simulink model "TST_FlWtDet_DD"  (R2016b)
settings: Solver=FixedStepDiscrete  StartTime=0.0  StopTime=simTime  FixedStep=sampleTime  RelTol=1e-3
values from neighbouring files (symbols this model uses):
  testCase = 1    [initTST_FlWtDet_DD_001.m]    (also in initTST_FlWtDet_DD_002.m = 2)
libraries: simulink x5, UnitTest_Lib x2
settings Model: Creator=zhengjinyan  LastModifiedBy=zhengjinyan
settings DebuggingCC: SignalRangeChecking=error

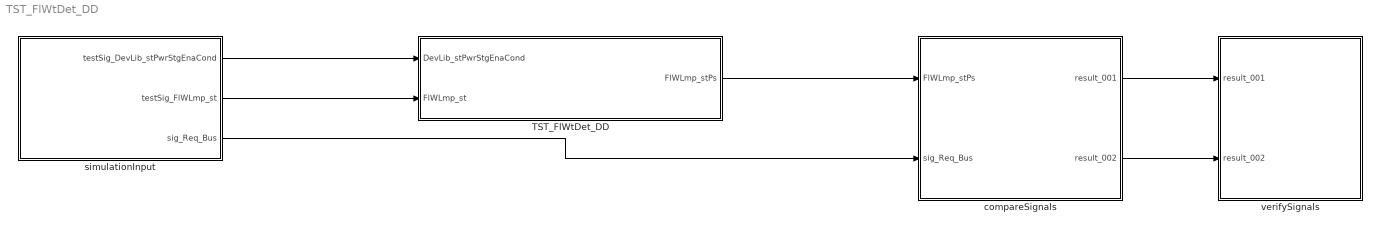
== system TST_FlWtDet_DD ==
  TST_FlWtDet_DD : Subsystem
  compareSignals : Subsystem
  simulationInput : Subsystem
  verifySignals : Subsystem
  wires:
  simulationInput/1(testSig_DevLib_stPwrStgEnaCond) -> TST_FlWtDet_DD/1(DevLib_stPwrStgEnaCond)
  simulationInput/2(testSig_FlWLmp_st) -> TST_FlWtDet_DD/2(FlWLmp_st)
  TST_FlWtDet_DD/1(FlWLmp_stPs) -> compareSignals/1(FlWLmp_stPs)
  simulationInput/3(sig_Req_Bus) -> compareSignals/2(sig_Req_Bus)
  compareSignals/1(result_001) -> verifySignals/1(result_001)
  compareSignals/2(result_002) -> verifySignals/2(result_002)

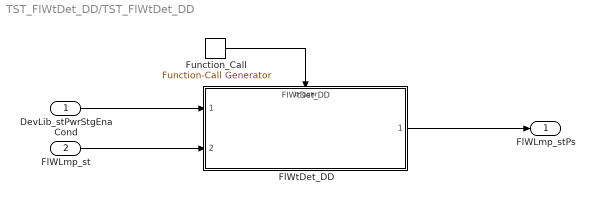
== system TST_FlWtDet_DD/TST_FlWtDet_DD ==
  DevLib_stPwrStgEnaCond : Inport
  FlWLmp_st : Inport  Port=2
  FlWtDet_DD : ModelReference  ModelNameDialog=FlWtDet_DD  SimulationMode=Normal  ModelReferenceVersion=1.8  TriggerPortName=function  TriggerPortTriggerType=function-call  TriggerPortStatesWhenEnabling=held
  Function_Call : simulink/Ports & Subsystems/Function-Call Generator  sample_time=sampleTime  numberOfIterations=1
  FlWLmp_stPs : Outport
  wires:
  Function_Call/1 -> FlWtDet_DD/Trigger
  DevLib_stPwrStgEnaCond/1 -> FlWtDet_DD/1
  FlWLmp_st/1 -> FlWtDet_DD/2
  FlWtDet_DD/1 -> FlWLmp_stPs/1

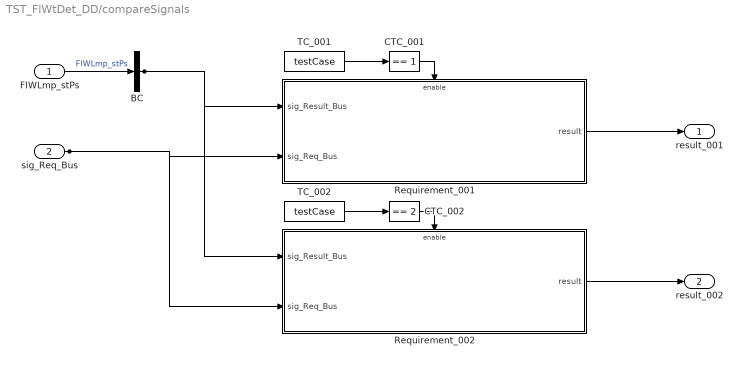
== system TST_FlWtDet_DD/compareSignals ==
  FlWLmp_stPs : Inport
  sig_Req_Bus : Inport  Port=2
  BC : BusCreator  Inputs=1
  CTC_001 : simulink/Logic and Bit Operations/Compare To Constant  relop===  const=1  OutDataTypeStr=boolean
  CTC_002 : simulink/Logic and Bit Operations/Compare To Constant  relop===  const=2  OutDataTypeStr=boolean
  Requirement_001 : Subsystem
  Requirement_002 : Subsystem
  TC_001 : Constant  Value=testCase
  TC_002 : Constant  Value=testCase
  result_001 : Outport
  result_002 : Outport  Port=2
  wires:
  FlWLmp_stPs/1 -> BC/1  "FlWLmp_stPs"
  TC_001/1 -> CTC_001/1
  CTC_001/1 -> Requirement_001/Enable
  sig_Req_Bus/1 -> Requirement_001/2(sig_Req_Bus), Requirement_002/2(sig_Req_Bus)
  BC/1 -> Requirement_001/1(sig_Result_Bus), Requirement_002/1(sig_Result_Bus)
  Requirement_001/1(result) -> result_001/1
  TC_002/1 -> CTC_002/1
  CTC_002/1 -> Requirement_002/Enable
  Requirement_002/1(result) -> result_002/1

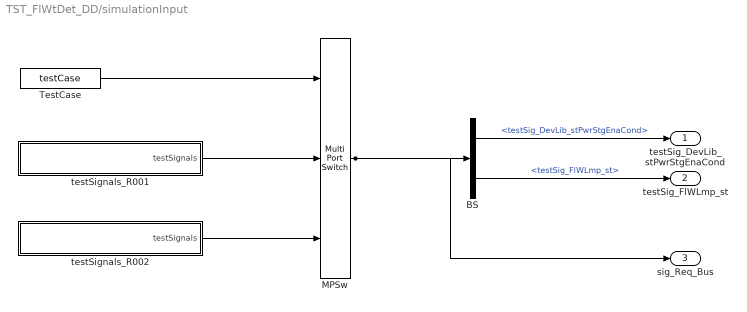
== system TST_FlWtDet_DD/simulationInput ==
  BS : BusSelector  OutputSignals=testSig_DevLib_stPwrStgEnaCond,testSig_FlWLmp_st
  MPSw : MultiPortSwitch  Inputs=2  SaturateOnIntegerOverflow=on  InputSameDT=on
  TestCase : Constant  Value=testCase
  testSignals_R001 : Subsystem
  testSignals_R002 : Subsystem
  testSig_DevLib_stPwrStgEnaCond : Outport
  testSig_FlWLmp_st : Outport  Port=2
  sig_Req_Bus : Outport  Port=3
  wires:
  BS/1 -> testSig_DevLib_stPwrStgEnaCond/1  "<testSig_DevLib_stPwrStgEnaCond>"
  BS/2 -> testSig_FlWLmp_st/1  "<testSig_FlWLmp_st>"
  MPSw/1 -> BS/1, sig_Req_Bus/1
  TestCase/1 -> MPSw/1
  testSignals_R001/1(testSignals) -> MPSw/2
  testSignals_R002/1(testSignals) -> MPSw/3

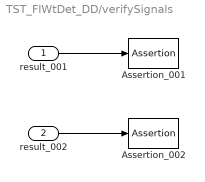
== system TST_FlWtDet_DD/verifySignals ==
  result_001 : Inport
  result_002 : Inport  Port=2
  Assertion_001 : Assertion  Enabled=off
  Assertion_002 : Assertion  Enabled=off
  wires:
  result_001/1 -> Assertion_001/1
  result_002/1 -> Assertion_002/1

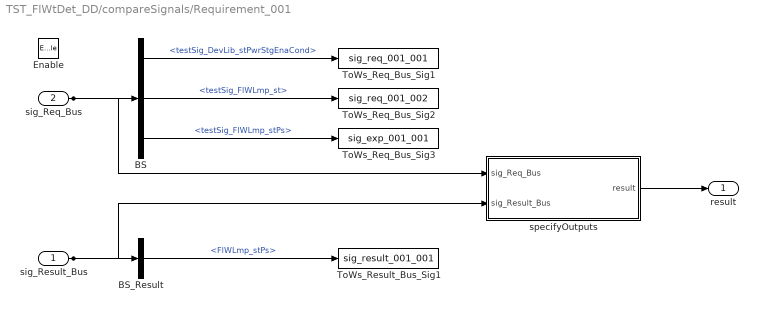
== system TST_FlWtDet_DD/compareSignals/Requirement_001 ==
  sig_Result_Bus : Inport
  sig_Req_Bus : Inport  Port=2
  Enable : EnablePort
  BS : BusSelector  OutputSignals=testSig_DevLib_stPwrStgEnaCond,testSig_FlWLmp_st,testSig_FlWLmp_stPs
  BS_Result : BusSelector  OutputSignals=FlWLmp_stPs
  ToWs_Req_Bus_Sig1 : ToWorkspace  VariableName=sig_req_001_001  SaveFormat=Structure With Time
  ToWs_Req_Bus_Sig2 : ToWorkspace  VariableName=sig_req_001_002  SaveFormat=Structure With Time
  ToWs_Req_Bus_Sig3 : ToWorkspace  VariableName=sig_exp_001_001  SaveFormat=Structure With Time
  ToWs_Result_Bus_Sig1 : ToWorkspace  VariableName=sig_result_001_001  SaveFormat=Structure With Time
  specifyOutputs : Subsystem
  result : Outport
  wires:
  sig_Req_Bus/1 -> BS/1, specifyOutputs/1(sig_Req_Bus)
  BS/1 -> ToWs_Req_Bus_Sig1/1  "<testSig_DevLib_stPwrStgEnaCond>"
  BS/2 -> ToWs_Req_Bus_Sig2/1  "<testSig_FlWLmp_st>"
  BS/3 -> ToWs_Req_Bus_Sig3/1  "<testSig_FlWLmp_stPs>"
  sig_Result_Bus/1 -> BS_Result/1, specifyOutputs/2(sig_Result_Bus)
  BS_Result/1 -> ToWs_Result_Bus_Sig1/1  "<FlWLmp_stPs>"
  specifyOutputs/1(result) -> result/1

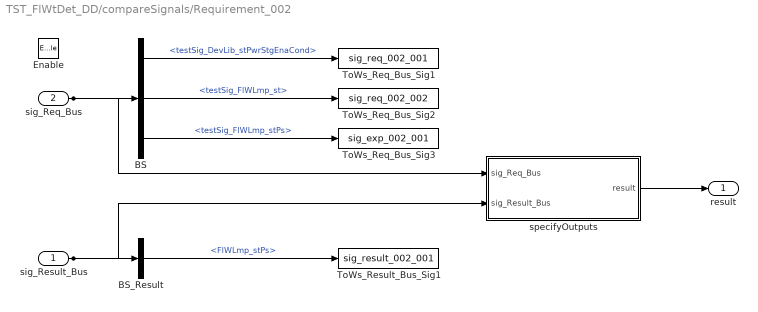
== system TST_FlWtDet_DD/compareSignals/Requirement_002 ==
  sig_Result_Bus : Inport
  sig_Req_Bus : Inport  Port=2
  Enable : EnablePort
  BS : BusSelector  OutputSignals=testSig_DevLib_stPwrStgEnaCond,testSig_FlWLmp_st,testSig_FlWLmp_stPs
  BS_Result : BusSelector  OutputSignals=FlWLmp_stPs
  ToWs_Req_Bus_Sig1 : ToWorkspace  VariableName=sig_req_002_001  SaveFormat=Structure With Time
  ToWs_Req_Bus_Sig2 : ToWorkspace  VariableName=sig_req_002_002  SaveFormat=Structure With Time
  ToWs_Req_Bus_Sig3 : ToWorkspace  VariableName=sig_exp_002_001  SaveFormat=Structure With Time
  ToWs_Result_Bus_Sig1 : ToWorkspace  VariableName=sig_result_002_001  SaveFormat=Structure With Time
  specifyOutputs : Subsystem
  result : Outport
  wires:
  sig_Req_Bus/1 -> BS/1, specifyOutputs/1(sig_Req_Bus)
  BS/1 -> ToWs_Req_Bus_Sig1/1  "<testSig_DevLib_stPwrStgEnaCond>"
  BS/2 -> ToWs_Req_Bus_Sig2/1  "<testSig_FlWLmp_st>"
  BS/3 -> ToWs_Req_Bus_Sig3/1  "<testSig_FlWLmp_stPs>"
  sig_Result_Bus/1 -> BS_Result/1, specifyOutputs/2(sig_Result_Bus)
  BS_Result/1 -> ToWs_Result_Bus_Sig1/1  "<FlWLmp_stPs>"
  specifyOutputs/1(result) -> result/1

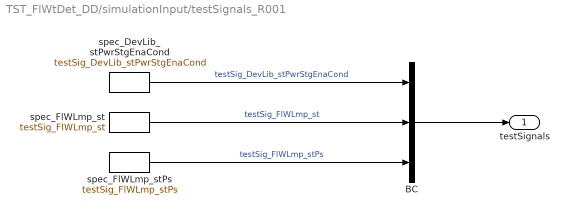
== system TST_FlWtDet_DD/simulationInput/testSignals_R001 ==
  BC : BusCreator  Inputs=3
  spec_DevLib_stPwrStgEnaCond : FromWorkspace  VariableName=testSig_DevLib_stPwrStgEnaCond  Interpolate=off  OutputAfterFinalValue=Holding final value
  spec_FlWLmp_st : FromWorkspace  VariableName=testSig_FlWLmp_st  Interpolate=off  OutputAfterFinalValue=Holding final value
  spec_FlWLmp_stPs : FromWorkspace  VariableName=testSig_FlWLmp_stPs  Interpolate=off  OutputAfterFinalValue=Holding final value
  testSignals : Outport
  wires:
  BC/1 -> testSignals/1
  spec_DevLib_stPwrStgEnaCond/1 -> BC/1  "testSig_DevLib_stPwrStgEnaCond"
  spec_FlWLmp_st/1 -> BC/2  "testSig_FlWLmp_st"
  spec_FlWLmp_stPs/1 -> BC/3  "testSig_FlWLmp_stPs"

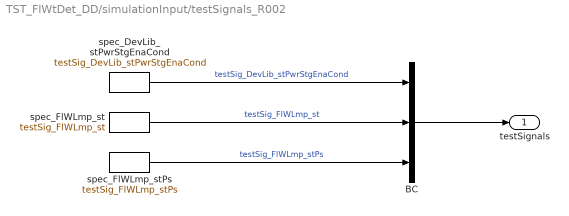
== system TST_FlWtDet_DD/simulationInput/testSignals_R002 ==
  BC : BusCreator  Inputs=3
  spec_DevLib_stPwrStgEnaCond : FromWorkspace  VariableName=testSig_DevLib_stPwrStgEnaCond  Interpolate=off  OutputAfterFinalValue=Holding final value
  spec_FlWLmp_st : FromWorkspace  VariableName=testSig_FlWLmp_st  Interpolate=off  OutputAfterFinalValue=Holding final value
  spec_FlWLmp_stPs : FromWorkspace  VariableName=testSig_FlWLmp_stPs  Interpolate=off  OutputAfterFinalValue=Holding final value
  testSignals : Outport
  wires:
  BC/1 -> testSignals/1
  spec_DevLib_stPwrStgEnaCond/1 -> BC/1  "testSig_DevLib_stPwrStgEnaCond"
  spec_FlWLmp_st/1 -> BC/2  "testSig_FlWLmp_st"
  spec_FlWLmp_stPs/1 -> BC/3  "testSig_FlWLmp_stPs"

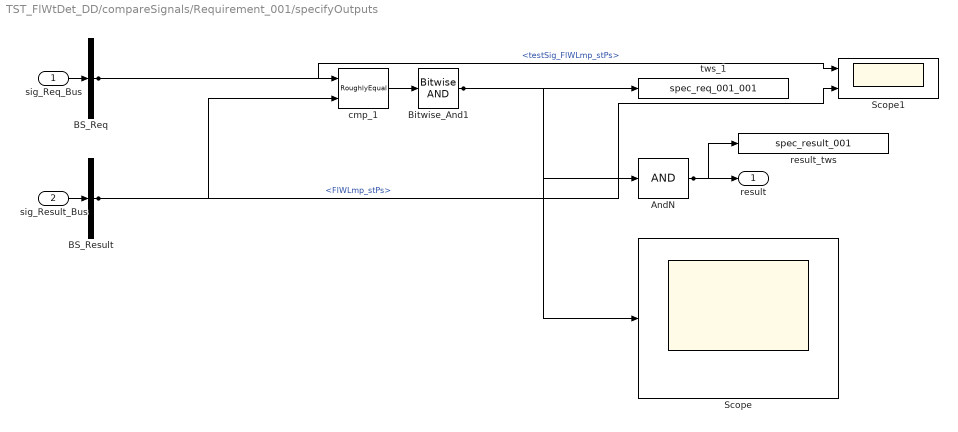
== system TST_FlWtDet_DD/compareSignals/Requirement_001/specifyOutputs ==
  sig_Req_Bus : Inport
  sig_Result_Bus : Inport  Port=2
  AndN : Logic  Inputs=1
  BS_Req : BusSelector  OutputSignals=testSig_FlWLmp_stPs
  BS_Result : BusSelector  OutputSignals=FlWLmp_stPs
  Bitwise_And1 : simulink/Logic and Bit Operations/Bitwise Operator  logicop=AND  UseBitMask=off  BitMask=bin2dec('11011001')  BitMaskRealWorld=Stored Integer
  Scope : Scope
  Scope1 : Scope  NumInputPorts=2
  cmp_1 : UnitTest_Lib/RoughlyEqual  slope=0.1
  result_tws : ToWorkspace  VariableName=spec_result_001
  tws_1 : ToWorkspace  VariableName=spec_req_001_001
  result : Outport
  wires:
  sig_Req_Bus/1 -> BS_Req/1
  sig_Result_Bus/1 -> BS_Result/1
  AndN/1 -> result/1, result_tws/1
  BS_Req/1 -> cmp_1/1, Scope1/1  "<testSig_FlWLmp_stPs>"
  BS_Result/1 -> cmp_1/2, Scope1/2  "<FlWLmp_stPs>"
  cmp_1/1 -> Bitwise_And1/1
  Bitwise_And1/1 -> tws_1/1, AndN/1, Scope/1

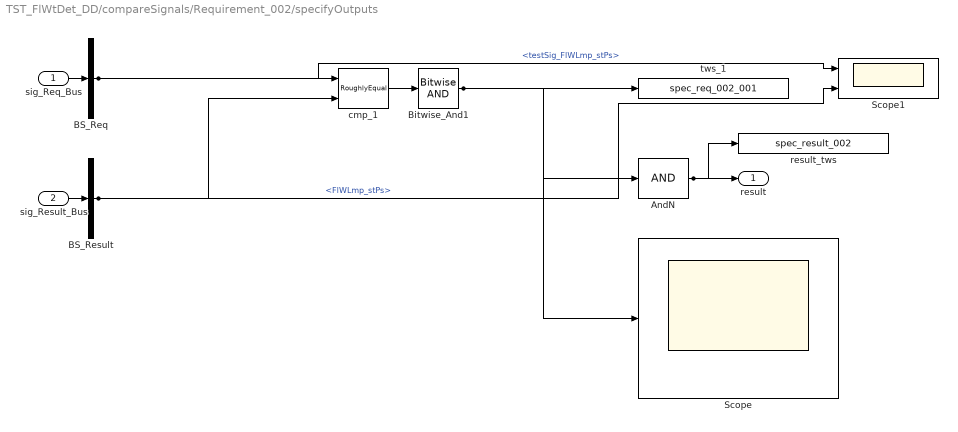
== system TST_FlWtDet_DD/compareSignals/Requirement_002/specifyOutputs ==
  sig_Req_Bus : Inport
  sig_Result_Bus : Inport  Port=2
  AndN : Logic  Inputs=1
  BS_Req : BusSelector  OutputSignals=testSig_FlWLmp_stPs
  BS_Result : BusSelector  OutputSignals=FlWLmp_stPs
  Bitwise_And1 : simulink/Logic and Bit Operations/Bitwise Operator  logicop=AND  UseBitMask=off  BitMask=bin2dec('11011001')  BitMaskRealWorld=Stored Integer
  Scope : Scope
  Scope1 : Scope  NumInputPorts=2
  cmp_1 : UnitTest_Lib/RoughlyEqual  slope=0.1
  result_tws : ToWorkspace  VariableName=spec_result_002
  tws_1 : ToWorkspace  VariableName=spec_req_002_001
  result : Outport
  wires:
  sig_Req_Bus/1 -> BS_Req/1
  sig_Result_Bus/1 -> BS_Result/1
  AndN/1 -> result/1, result_tws/1
  BS_Req/1 -> cmp_1/1, Scope1/1  "<testSig_FlWLmp_stPs>"
  BS_Result/1 -> cmp_1/2, Scope1/2  "<FlWLmp_stPs>"
  cmp_1/1 -> Bitwise_And1/1
  Bitwise_And1/1 -> tws_1/1, AndN/1, Scope/1
